simulink model "LKATestBenchExampleRL"  (R2020b)
settings: Solver=VariableStepAuto  StartTime=0.0  StopTime=simStopTime  RelTol=1e-3
PostLoadFcn:
  | helperLKASetUp
undefined symbols (not defined in the file): Curvature, CurvatureDerivative, DiscIntNeverNeededParam, driving, HeadingAngle, LateralOffset, Left, lr, m, PredictionHorizon, Right, Strength, Ts, v0_ego, yaw0_ego
libraries: simulink x4, drivingscenarioandsensors x2, mpcadaslib x1, rllib x1, autolibshared x1
CloseFcn:
  | helperLKACleanUp
settings Model: Creator=The MathWorks, Inc.  LastModifiedBy=adelicia
settings DataIOCC: ReturnWorkspaceOutputs=off
settings DebuggingCC: ParameterPrecisionLossMsg=none  ArithmeticOperatorsInVariantConditions=warning
settings HardwareCC: ProdLongLongMode=on
settings SFSimCC: SimUseLocalCustomCode=off
settings RTWCC: RTWUseLocalCustomCode=off

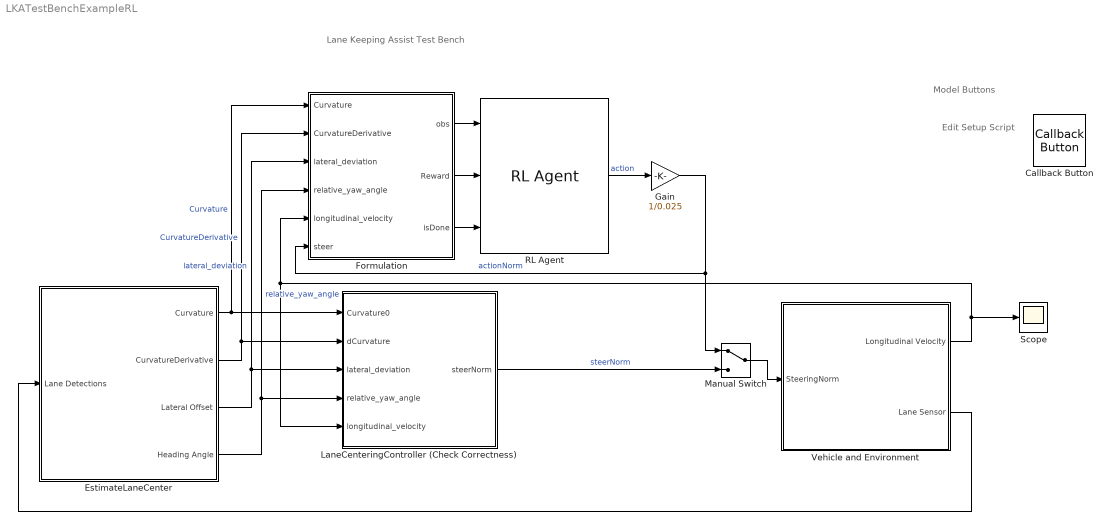
== system LKATestBenchExampleRL ==
  note: Edit Setup Script
  note: Lane Keeping Assist Test Bench
  note: Model Buttons
  Callback Button : CallbackButton  ButtonText=?
      settings: ClickFcn=|
      | exampleID = 'LaneKeepingAssistWithLaneDetectionExample';
      | exampleName = 'lane-keeping-assist-with-lane-detection.html';
      | if license('test','automated_driving_toolbox') && ~isempty(ver('driving'))
      |     helpview('driving',exampleID);
      | elseif license('test','MPC_Toolbox') && ~isempty(ver('mpc'))
      |     helpview('mpc',exampleID);
      | else
      |     web(fullfile('https://www.mathworks.com/help','driving','examples',exampleName));
      | end
      | clear exampleName exampleID;
  EstimateLaneCenter : Subsystem  VariantControl=v2
  Formulation : Subsystem
  Gain : Gain  Gain=1/0.025
  LaneCenteringController (Check Correctness) : Subsystem
  Manual Switch : ManualSwitch
  RL Agent : rllib/RL Agent  Agent=agent  ProvideReward=on  ProvideIsDone=on  ProvideCumRwd=off  TreatAsDirectFeedthrough=on  CollectLoggedSignals=on  CollectModelStates=on
  Scope : Scope
  Vehicle and Environment : Subsystem
  wires:
  Vehicle and Environment/2(Lane Sensor) -> EstimateLaneCenter/1(Lane Detections)
  EstimateLaneCenter/2(CurvatureDerivative) -> Formulation/2(CurvatureDerivative), LaneCenteringController (Check Correctness)/2(dCurvature)  "CurvatureDerivative"
  EstimateLaneCenter/3(Lateral Offset) -> Formulation/3(lateral_deviation), LaneCenteringController (Check Correctness)/3(lateral_deviation)  "lateral_deviation"
  EstimateLaneCenter/4(Heading Angle) -> Formulation/4(relative_yaw_angle), LaneCenteringController (Check Correctness)/4(relative_yaw_angle)  "relative_yaw_angle"
  Vehicle and Environment/1(Longitudinal Velocity) -> Scope/1, LaneCenteringController (Check Correctness)/5(longitudinal_velocity), Formulation/5(longitudinal_velocity)
  EstimateLaneCenter/1(Curvature) -> Formulation/1(Curvature), LaneCenteringController (Check Correctness)/1(Curvature0)  "Curvature"
  Formulation/1(obs) -> RL Agent/1
  Formulation/2(Reward) -> RL Agent/2
  Formulation/3(isDone) -> RL Agent/3
  LaneCenteringController (Check Correctness)/1(steerNorm) -> Manual Switch/2  "steerNorm"
  RL Agent/1 -> Gain/1  "action"
  Gain/1 -> Manual Switch/1, Formulation/6(steer)  "actionNorm"
  Manual Switch/1 -> Vehicle and Environment/1(SteeringNorm)

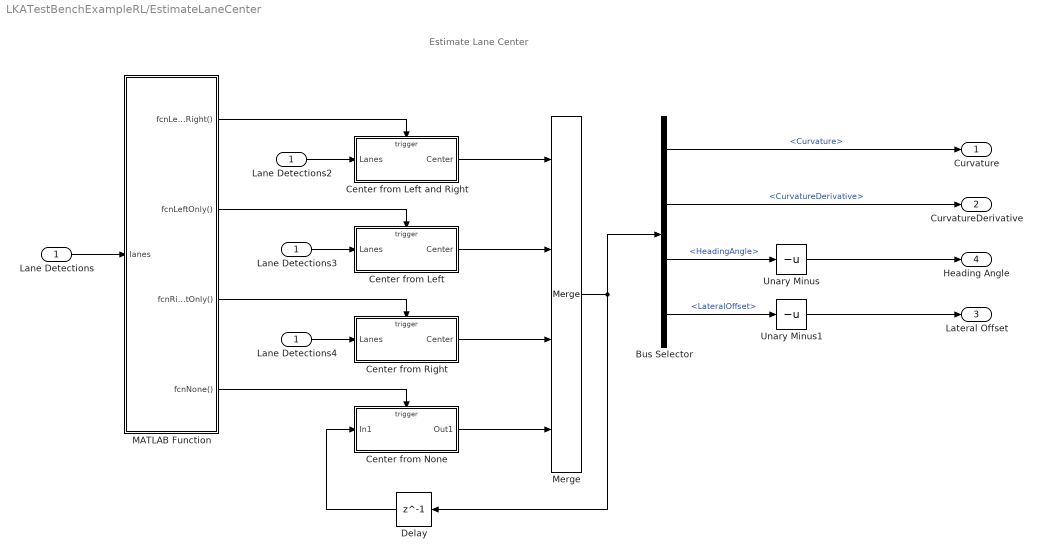
== system LKATestBenchExampleRL/EstimateLaneCenter ==
  note: Estimate Lane Center
  Lane Detections : Inport
  Bus Selector : BusSelector  OutputSignals=Curvature,CurvatureDerivative,HeadingAngle,LateralOffset
  Center from Left : Subsystem  TreatAsAtomicUnit=on
  Center from Left and Right : Subsystem  TreatAsAtomicUnit=on
  Center from None : Subsystem  TreatAsAtomicUnit=on
  Center from Right : Subsystem  TreatAsAtomicUnit=on
  Delay : Delay  DelayLength=1
  Lane Detections2 : InportShadow
  Lane Detections3 : InportShadow
  Lane Detections4 : InportShadow
  MATLAB Function : MATLAB Function  TreatAsAtomicUnit=on
  Merge : Merge  Inputs=4
  Unary Minus : UnaryMinus
  Unary Minus1 : UnaryMinus
  Curvature : Outport  VectorParamsAs1DForOutWhenUnconnected=off
  CurvatureDerivative : Outport  Port=2  VectorParamsAs1DForOutWhenUnconnected=off
  Lateral Offset : Outport  Port=3  VectorParamsAs1DForOutWhenUnconnected=off
  Heading Angle : Outport  Port=4  VectorParamsAs1DForOutWhenUnconnected=off
  wires:
  Bus Selector/3 -> Unary Minus/1  "<HeadingAngle>"
  Bus Selector/4 -> Unary Minus1/1  "<LateralOffset>"
  Bus Selector/1 -> Curvature/1  "<Curvature>"
  Bus Selector/2 -> CurvatureDerivative/1  "<CurvatureDerivative>"
  Unary Minus1/1 -> Lateral Offset/1
  Unary Minus/1 -> Heading Angle/1
  Merge/1 -> Delay/1, Bus Selector/1
  Center from Left/1(Center) -> Merge/2
  MATLAB Function/4(fcnNone()) -> Center from None/Trigger
  MATLAB Function/3(fcnRightOnly()) -> Center from Right/Trigger
  Lane Detections2/1 -> Center from Left and Right/1(Lanes)
  Lane Detections/1 -> MATLAB Function/1(lanes)
  Center from Left and Right/1(Center) -> Merge/1
  Delay/1 -> Center from None/1(In1)
  MATLAB Function/1(fcnLeftAndRight()) -> Center from Left and Right/Trigger
  Center from None/1(Out1) -> Merge/4
  MATLAB Function/2(fcnLeftOnly()) -> Center from Left/Trigger
  Lane Detections4/1 -> Center from Right/1(Lanes)
  Lane Detections3/1 -> Center from Left/1(Lanes)
  Center from Right/1(Center) -> Merge/3

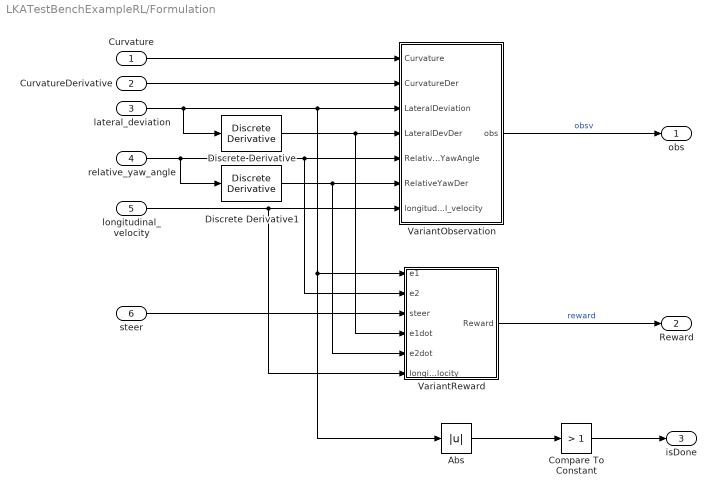
== system LKATestBenchExampleRL/Formulation ==
  Curvature : Inport
  CurvatureDerivative : Inport  Port=2
  lateral_deviation : Inport  Port=3
  relative_yaw_angle : Inport  Port=4
  longitudinal_velocity : Inport  Port=5
  steer : Inport  Port=6
  Abs : Abs
  Compare To Constant : simulink/Logic and Bit Operations/Compare To Constant  relop=>  const=1  OutDataTypeStr=boolean
  Discrete Derivative : simulink/Discrete/Discrete Derivative  gainval=1.0  ICPrevScaledInput=0.0  OutMin=[]  OutMax=[]  OutDataType=fixdt(1, 16)  OutScaling=2^-10  DoSatur=off
  Discrete Derivative1 : simulink/Discrete/Discrete Derivative  gainval=1.0  ICPrevScaledInput=0.0  OutMin=[]  OutMax=[]  OutDataType=fixdt(1, 16)  OutScaling=2^-10  DoSatur=off
  VariantObservation : Subsystem  Variant=on
  VariantReward : Subsystem  Variant=on
  obs : Outport
  Reward : Outport  Port=2  VectorParamsAs1DForOutWhenUnconnected=off
  isDone : Outport  Port=3  VectorParamsAs1DForOutWhenUnconnected=off
  wires:
  Curvature/1 -> VariantObservation/1(Curvature)
  CurvatureDerivative/1 -> VariantObservation/2(CurvatureDer)
  relative_yaw_angle/1 -> Discrete Derivative1/1, VariantReward/2(e2), VariantObservation/5(RelativeYawAngle)
  VariantObservation/1(obs) -> obs/1  "obsv"
  steer/1 -> VariantReward/3(steer)
  VariantReward/1(Reward) -> Reward/1  "reward"
  lateral_deviation/1 -> Discrete Derivative/1, Abs/1, VariantReward/1(e1), VariantObservation/3(LateralDeviation)
  Abs/1 -> Compare To Constant/1
  Compare To Constant/1 -> isDone/1
  Discrete Derivative/1 -> VariantReward/4(e1dot), VariantObservation/4(LateralDevDer)
  Discrete Derivative1/1 -> VariantReward/5(e2dot), VariantObservation/6(RelativeYawDer)
  longitudinal_velocity/1 -> VariantReward/6(longitudinal_velocity), VariantObservation/7(longitudinal_velocity)

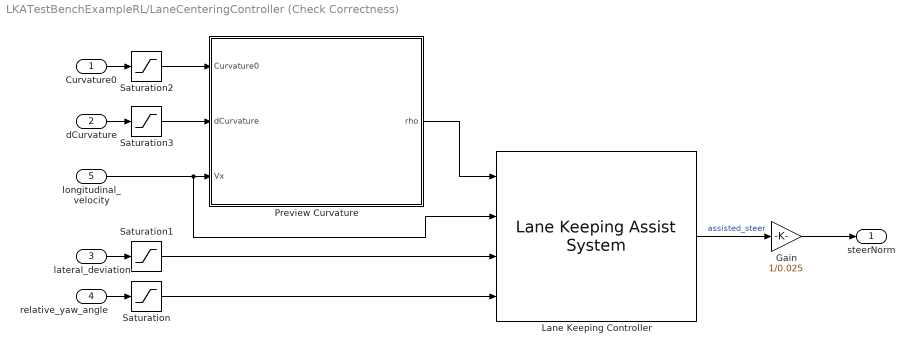
== system LKATestBenchExampleRL/LaneCenteringController (Check Correctness) ==
  Curvature0 : Inport
  dCurvature : Inport  Port=2
  lateral_deviation : Inport  Port=3
  relative_yaw_angle : Inport  Port=4
  longitudinal_velocity : Inport  Port=5
  Gain : Gain  Gain=1/0.025
  Lane Keeping Controller : mpcadaslib/Lane Keeping Assist System  ModelType=Use vehicle parameters  VehicleMass=m  VehicleYawInertia=Iz  LengthToFront=lf  LengthToRear=lr  FrontTireStiffness=Cf  RearTireStiffness=Cr  EgoModelMatrixA=[-4.4021 ,-12.4603;1.3913,-5.1868]  EgoModelMatrixB=[24.1270;15.8609]  EgoModelMatrixC=[1,0;0,1]  InitialLongVel=v0_ego  TransportLag=0  MinSteering=-0.5  umin_ext=off  MaxSteering=0.5  umax_ext=off  Ts=Ts  PredictionHorizon=PredictionHorizon  ControllerBehavior=0.200  suboptimal=off  maxiter=10  datatypeopt=single  optmode=off  trackmode=off
      settings: SourceProductBaseCode=MP
  Preview Curvature : MATLAB Function  TreatAsAtomicUnit=on  SystemSampleTime=Ts
  Saturation : Saturate
  Saturation1 : Saturate  UpperLimit=0.6  LowerLimit=-0.6
  Saturation2 : Saturate  UpperLimit=0.15  LowerLimit=-0.15
  Saturation3 : Saturate  UpperLimit=0.06  LowerLimit=-0.06
  steerNorm : Outport
  wires:
  relative_yaw_angle/1 -> Saturation/1
  dCurvature/1 -> Saturation3/1
  Preview Curvature/1(rho) -> Lane Keeping Controller/1
  longitudinal_velocity/1 -> Lane Keeping Controller/2, Preview Curvature/3(Vx)
  Curvature0/1 -> Saturation2/1
  lateral_deviation/1 -> Saturation1/1
  Saturation2/1 -> Preview Curvature/1(Curvature0)
  Saturation3/1 -> Preview Curvature/2(dCurvature)
  Saturation1/1 -> Lane Keeping Controller/3
  Saturation/1 -> Lane Keeping Controller/4
  Lane Keeping Controller/1 -> Gain/1  "assisted_steer"
  Gain/1 -> steerNorm/1

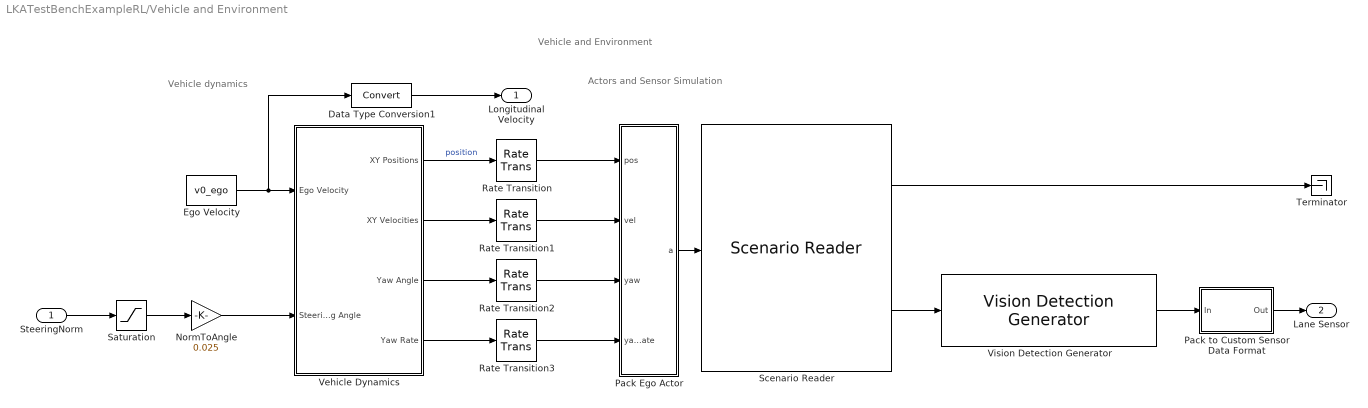
== system LKATestBenchExampleRL/Vehicle and Environment ==
  note: Vehicle dynamics
  note: Actors and Sensor Simulation
  note: Vehicle and Environment
  SteeringNorm : Inport  Unit=rad
  Data Type Conversion1 : DataTypeConversion
  Ego Velocity : Constant  Value=v0_ego  SampleTime=Ts
  NormToAngle : Gain  Gain=0.025
  Pack Ego Actor : MATLAB Function  TreatAsAtomicUnit=on
  Pack to Custom Sensor Data Format : Subsystem
  Rate Transition{,1..3} (4 alike) : RateTransition  OutPortSampleTime=Ts
  Saturation : Saturate  UpperLimit=1  LowerLimit=-1
  Scenario Reader : drivingscenarioandsensors/Scenario Reader  ScenarioSource=From workspace  ScenarioFileName=LKATestBenchScenario.mat  ScenarioVariableName=scenario  OutputCoordinateSystem=Vehicle coordinates  EgoVehicleSource=Input port  EgoVehicleActorID=1  OrientVehiclesOnRoad=off  OutputEgoVehiclePose=off  SampleTime=0.1  LaneBoundaryOutput=Ego vehicle lane boundaries  LaneBoundaryDistance=0:0.5:60  LaneBoundaryLocation=Inner edge of lane markings  BusNameSource=Auto  BusName=BusActors  BusName2Source=Auto  BusName2=BusLaneBoundaries  BusName3Source=Auto  BusName3=BusEgoActor  ShowCoordinateLabels=on  SimulateUsing=Interpreted execution
  Terminator : Terminator
  Vehicle Dynamics : Subsystem  VariantControl=VariantVDBS
  Vision Detection Generator : drivingscenarioandsensors/Vision Detection Generator  SensorIndex=1  DetectorOutput=Lanes only  UpdateInterval=0.1  LaneUpdateInterval=0.1  SensorLocation=[ 1.9, 0 ]  Height=1.1  Yaw=0  Pitch=1  Roll=0  BusNameSource=Auto  BusName=BusObjectDetections  BusName2Source=Property  BusName2=BusVision  MaxNumDetectionsSource=Property  MaxNumDetections=50  MaxNumLanesSource=Property  MaxNumLanes=2  DetectionCoordinates=Ego Cartesian  SimulateUsing=Interpreted execution  MaxRange=150  BoundingBoxAccuracy=5  ProcessNoiseIntensity=5  MaxSpeed=50  MaxAllowedOcclusion=0.5  MinObjectImageSize=[ 15, 15 ]  DetectionProbability=0.9  FalsePositivesPerImage=0.1  MinLaneImageSize=[ 20, 3 ]  LaneBoundaryAccuracy=3  HasNoise=on  InitialSeedSource=Repeatable  InitialSeed=0  UsedSeed=driving.internal.SimulinkUtilities.seedManager(gcb)  ActorProfilesSource=Parameters  ActorProfilesParameters=driving.internal.ActorProfilesParameters  ActorProfilesExpression=struct( 'ClassID', 0, 'Length', 4.7, 'Width', 1.8, 'Height', 1.4, 'OriginOffset', [ -1.35, 0, 0 ] )  Intrinsics=driving.internal.cameraIntrinsics
  Longitudinal Velocity : Outport  OutDataTypeStr=single  Unit=m/s  VectorParamsAs1DForOutWhenUnconnected=off
  Lane Sensor : Outport  Port=2  VectorParamsAs1DForOutWhenUnconnected=off
  wires:
  Ego Velocity/1 -> Data Type Conversion1/1, Vehicle Dynamics/1(Ego Velocity)
  Scenario Reader/1 -> Terminator/1
  Pack Ego Actor/1(a) -> Scenario Reader/1
  Vehicle Dynamics/2(XY Velocities) -> Rate Transition1/1
  Vehicle Dynamics/3(Yaw Angle) -> Rate Transition2/1
  Rate Transition/1 -> Pack Ego Actor/1(pos)
  Vehicle Dynamics/4(Yaw Rate) -> Rate Transition3/1
  Rate Transition2/1 -> Pack Ego Actor/3(yaw)
  Rate Transition1/1 -> Pack Ego Actor/2(vel)
  Rate Transition3/1 -> Pack Ego Actor/4(yawRate)
  Scenario Reader/2 -> Vision Detection Generator/1
  Vehicle Dynamics/1(XY Positions) -> Rate Transition/1  "position"
  Vision Detection Generator/1 -> Pack to Custom Sensor Data Format/1(In)
  Pack to Custom Sensor Data Format/1(Out) -> Lane Sensor/1
  Data Type Conversion1/1 -> Longitudinal Velocity/1
  SteeringNorm/1 -> Saturation/1
  NormToAngle/1 -> Vehicle Dynamics/2(Steering Angle)
  Saturation/1 -> NormToAngle/1

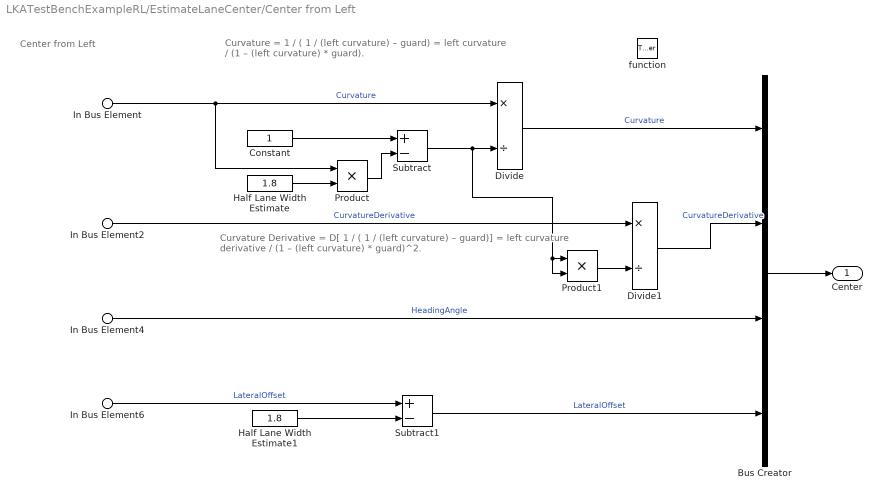
== system LKATestBenchExampleRL/EstimateLaneCenter/Center from Left ==
  note: Curvature
      | = 1 / ( 1 / (left curvature) – guard)
      | = left curvature / (1 – (left curvature) * guard).
  note: Center from Left
  note: Curvature Derivative
      | = D[ 1 / ( 1 / (left curvature) – guard)]
      | = left curvature derivative / (1 – (left curvature) * guard)^2.
  In Bus Element : Inport  PortName=Lanes  Element=Left.Curvature
  In Bus Element2 : Inport  PortName=Lanes  Element=Left.CurvatureDerivative
  In Bus Element4 : Inport  PortName=Lanes  Element=Left.HeadingAngle
  In Bus Element6 : Inport  PortName=Lanes  Element=Left.LateralOffset
  function : TriggerPort  TriggerType=function-call  VariantControl=Variant
  Bus Creator : BusCreator  Inputs=4
  Constant : Constant  OutDataTypeStr=Inherit: Inherit via back propagation
  Divide : Product  Inputs=*/
  Divide1 : Product  Inputs=*/
  Half Lane Width Estimate : Constant  Value=1.8  OutDataTypeStr=Inherit: Inherit via back propagation
  Half Lane Width Estimate1 : Constant  Value=1.8  OutDataTypeStr=Inherit: Inherit via back propagation
  Product : Product
  Product1 : Product
  Subtract : Sum  Inputs=+-
  Subtract1 : Sum  Inputs=+-
  Center : Outport  VectorParamsAs1DForOutWhenUnconnected=off
  wires:
  Bus Creator/1 -> Center/1
  Divide1/1 -> Bus Creator/2  "CurvatureDerivative"
  Divide/1 -> Bus Creator/1  "Curvature"
  In Bus Element4/1 -> Bus Creator/3  "HeadingAngle"
  Subtract1/1 -> Bus Creator/4  "LateralOffset"
  In Bus Element/1 -> Product/1, Divide/1  "Curvature"
  Subtract/1 -> Product1/2, Product1/1, Divide/2
  Half Lane Width Estimate/1 -> Product/2
  Constant/1 -> Subtract/1
  In Bus Element2/1 -> Divide1/1  "CurvatureDerivative"
  Product1/1 -> Divide1/2
  In Bus Element6/1 -> Subtract1/1  "LateralOffset"
  Half Lane Width Estimate1/1 -> Subtract1/2
  Product/1 -> Subtract/2

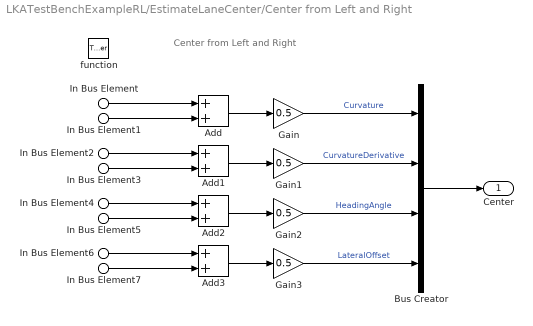
== system LKATestBenchExampleRL/EstimateLaneCenter/Center from Left and Right ==
  note: Center from Left and Right
  In Bus Element : Inport  PortName=Lanes  Element=Left.Curvature
  In Bus Element2 : Inport  PortName=Lanes  Element=Left.CurvatureDerivative
  In Bus Element4 : Inport  PortName=Lanes  Element=Left.HeadingAngle
  In Bus Element6 : Inport  PortName=Lanes  Element=Left.LateralOffset
  In Bus Element1 : Inport  PortName=Lanes  Element=Right.Curvature
  In Bus Element3 : Inport  PortName=Lanes  Element=Right.CurvatureDerivative
  In Bus Element5 : Inport  PortName=Lanes  Element=Right.HeadingAngle
  In Bus Element7 : Inport  PortName=Lanes  Element=Right.LateralOffset
  function : TriggerPort  TriggerType=function-call  VariantControl=Variant
  Add{,1..3} (4 alike) : Sum
  Bus Creator : BusCreator  Inputs=4
  Gain{,1..3} (4 alike) : Gain  Gain=0.5
  Center : Outport  VectorParamsAs1DForOutWhenUnconnected=off
  wires:
  Add/1 -> Gain/1
  Gain/1 -> Bus Creator/1  "Curvature"
  Add1/1 -> Gain1/1
  Gain1/1 -> Bus Creator/2  "CurvatureDerivative"
  Add2/1 -> Gain2/1
  Gain2/1 -> Bus Creator/3  "HeadingAngle"
  Add3/1 -> Gain3/1
  Gain3/1 -> Bus Creator/4  "LateralOffset"
  Bus Creator/1 -> Center/1
  In Bus Element/1 -> Add/1
  In Bus Element1/1 -> Add/2
  In Bus Element2/1 -> Add1/1
  In Bus Element3/1 -> Add1/2
  In Bus Element4/1 -> Add2/1
  In Bus Element5/1 -> Add2/2
  In Bus Element7/1 -> Add3/2
  In Bus Element6/1 -> Add3/1

== system LKATestBenchExampleRL/EstimateLaneCenter/Center from None ==
  In1 : Inport
  function : TriggerPort  TriggerType=function-call  VariantControl=Variant
  Out1 : Outport  VectorParamsAs1DForOutWhenUnconnected=off
  wires:
  In1/1 -> Out1/1

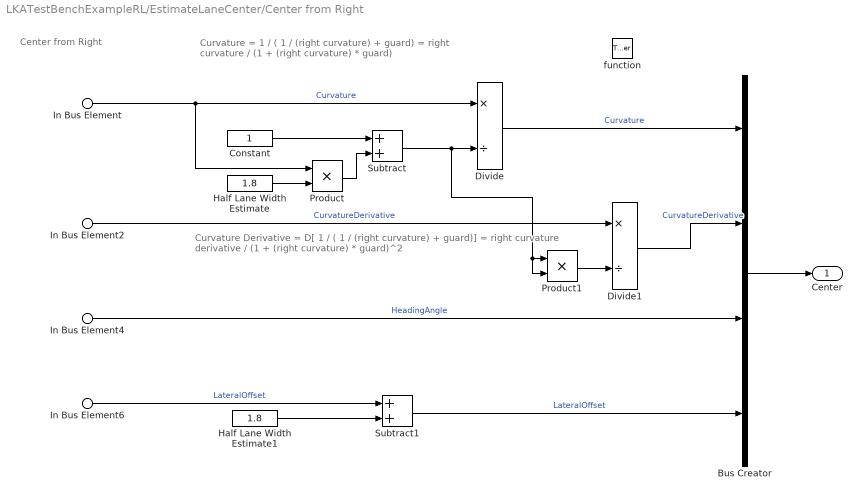
== system LKATestBenchExampleRL/EstimateLaneCenter/Center from Right ==
  note: Center from Right
  note: Curvature
      | = 1 / ( 1 / (right curvature) + guard)
      | = right curvature / (1 + (right curvature) * guard)
  note: Curvature Derivative
      | = D[ 1 / ( 1 / (right curvature) + guard)]
      | = right curvature derivative / (1 + (right curvature) * guard)^2
  In Bus Element : Inport  PortName=Lanes  Element=Right.Curvature
  In Bus Element2 : Inport  PortName=Lanes  Element=Right.CurvatureDerivative
  In Bus Element4 : Inport  PortName=Lanes  Element=Right.HeadingAngle
  In Bus Element6 : Inport  PortName=Lanes  Element=Right.LateralOffset
  function : TriggerPort  TriggerType=function-call  VariantControl=Variant
  Bus Creator : BusCreator  Inputs=4
  Constant : Constant  OutDataTypeStr=Inherit: Inherit via back propagation
  Divide : Product  Inputs=*/
  Divide1 : Product  Inputs=*/
  Half Lane Width Estimate : Constant  Value=1.8  OutDataTypeStr=Inherit: Inherit via back propagation
  Half Lane Width Estimate1 : Constant  Value=1.8  OutDataTypeStr=Inherit: Inherit via back propagation
  Product : Product
  Product1 : Product
  Subtract : Sum
  Subtract1 : Sum
  Center : Outport  VectorParamsAs1DForOutWhenUnconnected=off
  wires:
  In Bus Element2/1 -> Divide1/1  "CurvatureDerivative"
  Divide1/1 -> Bus Creator/2  "CurvatureDerivative"
  Product1/1 -> Divide1/2
  In Bus Element4/1 -> Bus Creator/3  "HeadingAngle"
  Half Lane Width Estimate1/1 -> Subtract1/2
  In Bus Element6/1 -> Subtract1/1  "LateralOffset"
  Divide/1 -> Bus Creator/1  "Curvature"
  Subtract1/1 -> Bus Creator/4  "LateralOffset"
  Bus Creator/1 -> Center/1
  In Bus Element/1 -> Product/1, Divide/1  "Curvature"
  Subtract/1 -> Product1/2, Product1/1, Divide/2
  Constant/1 -> Subtract/1
  Product/1 -> Subtract/2
  Half Lane Width Estimate/1 -> Product/2

== system LKATestBenchExampleRL/Formulation/VariantObservation ==
  note: 1) Add Subsystem or Model blocks as valid variant choices.
      | 2) You cannot connect blocks at this level. At simulation, connectivity is automatically
      | determined, based on the active variant and port name matching.
  Curvature : Inport
  CurvatureDer : Inport  Port=2
  LateralDeviation : Inport  Port=3
  LateralDevDer : Inport  Port=4
  RelativeYawAngle : Inport  Port=5
  RelativeYawDer : Inport  Port=6
  longitudinal_velocity : Inport  Port=7
  EightStates : Subsystem  VariantControl=OBSV_MODE_EIGHT
  FourStates : Subsystem  VariantControl=OBSV_MODE_FOUR
  TwoStates : Subsystem  VariantControl=OBSV_MODE_TWO
  obs : Outport

== system LKATestBenchExampleRL/Formulation/VariantReward ==
  note: 1) Add Subsystem or Model blocks as valid variant choices.
      | 2) You cannot connect blocks at this level. At simulation, connectivity is automatically
      | determined, based on the active variant and port name matching.
  e1 : Inport
  e2 : Inport  Port=2
  steer : Inport  Port=3
  e1dot : Inport  Port=4
  e2dot : Inport  Port=5
  longitudinal_velocity : Inport  Port=6
  QuardraticReward : Subsystem  VariantControl=REWARD_MODE_QUADRATIC
  TrgonometryReward : Subsystem  VariantControl=REWARD_MODE_TRIGONOMETRY
  Reward : Outport

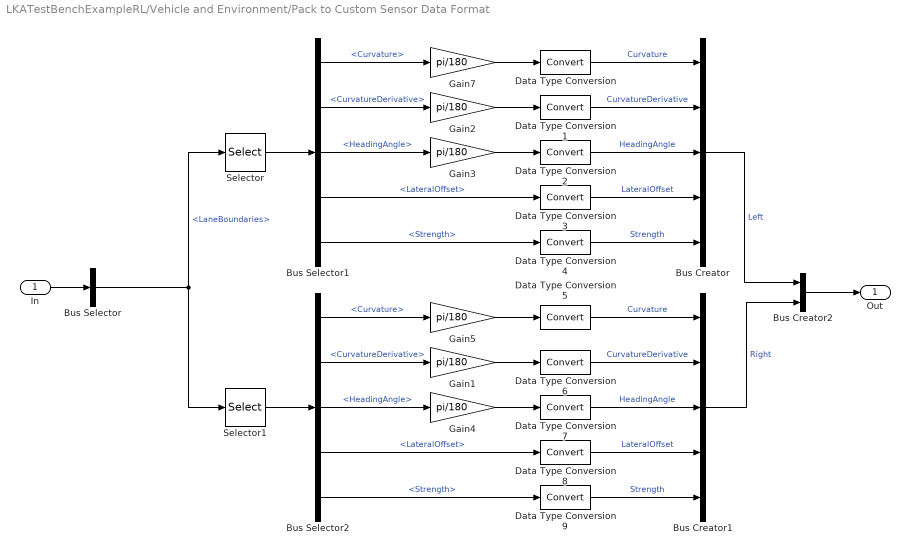
== system LKATestBenchExampleRL/Vehicle and Environment/Pack to Custom Sensor Data Format ==
  In : Inport
  Bus Creator : BusCreator  Inputs=Curvature,CurvatureDerivative,HeadingAngle,LateralOffset,Strength  OutDataTypeStr=Bus: LaneSensorBoundaries
  Bus Creator1 : BusCreator  Inputs=Curvature,CurvatureDerivative,HeadingAngle,LateralOffset,Strength  OutDataTypeStr=Bus: LaneSensorBoundaries
  Bus Creator2 : BusCreator  Inputs=Left,Right  OutDataTypeStr=Bus: LaneSensor
  Bus Selector : BusSelector  OutputSignals=LaneBoundaries
  Bus Selector1 : BusSelector  OutputSignals=Curvature,CurvatureDerivative,HeadingAngle,LateralOffset,Strength
  Bus Selector2 : BusSelector  OutputSignals=Curvature,CurvatureDerivative,HeadingAngle,LateralOffset,Strength
  Data Type Conversion{,1..9} (10 alike) : DataTypeConversion
  Gain{1..5,7} (6 alike) : Gain  Gain=pi/180
  Selector : Selector  InputPortWidth=2  IndexOptions=Index vector (dialog)  Indices=1  OutputSizes=1
  Selector1 : Selector  InputPortWidth=2  IndexOptions=Index vector (dialog)  Indices=2  OutputSizes=1
  Out : Outport  VectorParamsAs1DForOutWhenUnconnected=off
  wires:
  In/1 -> Bus Selector/1
  Bus Selector/1 -> Selector/1, Selector1/1  "<LaneBoundaries>"
  Selector/1 -> Bus Selector1/1
  Bus Selector1/2 -> Gain2/1  "<CurvatureDerivative>"
  Bus Selector1/1 -> Gain7/1  "<Curvature>"
  Bus Selector1/3 -> Gain3/1  "<HeadingAngle>"
  Gain7/1 -> Data Type Conversion/1
  Gain2/1 -> Data Type Conversion1/1
  Gain3/1 -> Data Type Conversion2/1
  Bus Selector1/4 -> Data Type Conversion3/1  "<LateralOffset>"
  Bus Selector1/5 -> Data Type Conversion4/1  "<Strength>"
  Data Type Conversion/1 -> Bus Creator/1  "Curvature"
  Data Type Conversion1/1 -> Bus Creator/2  "CurvatureDerivative"
  Data Type Conversion2/1 -> Bus Creator/3  "HeadingAngle"
  Data Type Conversion3/1 -> Bus Creator/4  "LateralOffset"
  Data Type Conversion4/1 -> Bus Creator/5  "Strength"
  Data Type Conversion9/1 -> Bus Creator1/5  "Strength"
  Data Type Conversion6/1 -> Bus Creator1/2  "CurvatureDerivative"
  Data Type Conversion7/1 -> Bus Creator1/3  "HeadingAngle"
  Data Type Conversion8/1 -> Bus Creator1/4  "LateralOffset"
  Data Type Conversion5/1 -> Bus Creator1/1  "Curvature"
  Bus Selector2/1 -> Gain5/1  "<Curvature>"
  Selector1/1 -> Bus Selector2/1
  Bus Selector2/4 -> Data Type Conversion8/1  "<LateralOffset>"
  Bus Selector2/5 -> Data Type Conversion9/1  "<Strength>"
  Bus Selector2/2 -> Gain1/1  "<CurvatureDerivative>"
  Gain4/1 -> Data Type Conversion7/1
  Gain5/1 -> Data Type Conversion5/1
  Gain1/1 -> Data Type Conversion6/1
  Bus Selector2/3 -> Gain4/1  "<HeadingAngle>"
  Bus Creator2/1 -> Out/1
  Bus Creator/1 -> Bus Creator2/1  "Left"
  Bus Creator1/1 -> Bus Creator2/2  "Right"

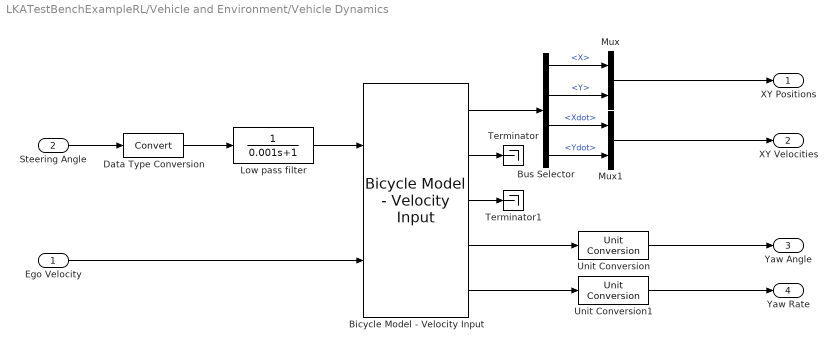
== system LKATestBenchExampleRL/Vehicle and Environment/Vehicle Dynamics ==
  Ego Velocity : Inport
  Steering Angle : Inport  Port=2
  Bicycle Model - Velocity Input : autolibshared/Bicycle Model - Velocity Input  trackMode=Single (bicycle)  inputMode=External longitudinal forces  frontSteerMode=on  rearSteerMode=off  windMode=off  muMode=off  extFMode=off  extMMode=off  aMode=3  NF=2  NR=2  m=m  a=lf  b=lr  h=0.35  X_o=x0_ego  xdot_o=0  CalphaMode=off  sigmaMode=on  w=[1.4,1.4]  Cy_f=Cf  Cy_r=Cr  sigma_f=.1  sigma_r=.1  alpha_f_brk=[-.1 .1]  Cy_f_data=[-9e3 9e3]  alpha_r_brk=[-.1 .1]  Cy_r_data=[-9e3 9e3]  Y_o=y0_ego  ydot_o=0  Izz=Iz  psi_o=yaw0_ego*pi/180  r_o=0  Af=2  Cd=.3  Cl=.1  Cpm=.1  beta_w=[0:0.01:0.3]  Cs=[0:0.03:0.9]  Cym=[0:0.01:0.3]  Pabs=101325  Tair=273  g=9.81  mu=1  xdot_tol=.01  Fznom=5000  Fxtire_sat=1e6  Fytire_sat=1e6  longOff=0  latOff=0  vertOff=0
      settings: SourceProductBaseCode=PW,MT,UV,VE,VP
  Bus Selector : BusSelector  OutputSignals=InertFrm.FrntAxl.Disp.X,InertFrm.FrntAxl.Disp.Y,InertFrm.FrntAxl.Vel.Xdot,InertFrm.FrntAxl.Vel.Ydot
  Data Type Conversion : DataTypeConversion
  Low pass filter : TransferFcn  Denominator=[0.001 1]
  Mux : Mux  Inputs=2
  Mux1 : Mux  Inputs=2
  Terminator : Terminator
  Terminator1 : Terminator
  Unit Conversion : UnitConversion  OutputType=Inherit: Inherit via back propagation
  Unit Conversion1 : UnitConversion  OutputType=Inherit: Inherit via back propagation
  XY Positions : Outport  Unit=m  VectorParamsAs1DForOutWhenUnconnected=off
  XY Velocities : Outport  Port=2  Unit=m/s  VectorParamsAs1DForOutWhenUnconnected=off
  Yaw Angle : Outport  Port=3  Unit=deg  VectorParamsAs1DForOutWhenUnconnected=off
  Yaw Rate : Outport  Port=4  Unit=degree/s  VectorParamsAs1DForOutWhenUnconnected=off
  wires:
  Mux/1 -> XY Positions/1
  Mux1/1 -> XY Velocities/1
  Unit Conversion1/1 -> Yaw Rate/1
  Unit Conversion/1 -> Yaw Angle/1
  Ego Velocity/1 -> Bicycle Model - Velocity Input/2
  Bicycle Model - Velocity Input/1 -> Bus Selector/1
  Bicycle Model - Velocity Input/2 -> Terminator/1
  Bicycle Model - Velocity Input/3 -> Terminator1/1
  Bicycle Model - Velocity Input/4 -> Unit Conversion/1
  Bicycle Model - Velocity Input/5 -> Unit Conversion1/1
  Bus Selector/1 -> Mux/1  "<X>"
  Bus Selector/2 -> Mux/2  "<Y>"
  Bus Selector/3 -> Mux1/1  "<Xdot>"
  Bus Selector/4 -> Mux1/2  "<Ydot>"
  Data Type Conversion/1 -> Low pass filter/1
  Steering Angle/1 -> Data Type Conversion/1
  Low pass filter/1 -> Bicycle Model - Velocity Input/1

== system LKATestBenchExampleRL/Formulation/VariantObservation/EightStates ==
  Curvature : Inport
  CurvatureDer : Inport  Port=2
  LateralDeviation : Inport  Port=3
  LateralDevDer : Inport  Port=4
  RelativeYawAngle : Inport  Port=5
  RelativeYawDer : Inport  Port=6
  longitudinal_velocity : Inport  Port=7
  Discrete-Time Integrator : DiscreteIntegrator  SampleTime=-1  ICPrevOutput=DiscIntNeverNeededParam  ICPrevScaledInput=DiscIntNeverNeededParam
  Discrete-Time Integrator1 : DiscreteIntegrator  SampleTime=-1  ICPrevOutput=DiscIntNeverNeededParam  ICPrevScaledInput=DiscIntNeverNeededParam
  Mux : Mux  Inputs=8
  Terminator : Terminator
  obs : Outport  VectorParamsAs1DForOutWhenUnconnected=off
  wires:
  Mux/1 -> obs/1
  CurvatureDer/1 -> Mux/2
  Curvature/1 -> Mux/1
  LateralDeviation/1 -> Discrete-Time Integrator1/1, Mux/3
  Discrete-Time Integrator1/1 -> Mux/4  "integral_error"
  RelativeYawAngle/1 -> Discrete-Time Integrator/1, Mux/6
  Discrete-Time Integrator/1 -> Mux/7  "integral_error"
  LateralDevDer/1 -> Mux/5
  RelativeYawDer/1 -> Mux/8
  longitudinal_velocity/1 -> Terminator/1

== system LKATestBenchExampleRL/Formulation/VariantObservation/FourStates ==
  Curvature : Inport
  CurvatureDer : Inport  Port=2
  LateralDeviation : Inport  Port=3
  LateralDevDer : Inport  Port=4
  RelativeYawAngle : Inport  Port=5
  RelativeYawDer : Inport  Port=6
  longitudinal_velocity : Inport  Port=7
  Mux : Mux
  Terminator1 : Terminator
  Terminator2 : Terminator
  Terminator3 : Terminator
  obs : Outport  VectorParamsAs1DForOutWhenUnconnected=off
  wires:
  Mux/1 -> obs/1
  Curvature/1 -> Mux/1
  CurvatureDer/1 -> Mux/2
  LateralDevDer/1 -> Terminator1/1
  RelativeYawDer/1 -> Terminator2/1
  RelativeYawAngle/1 -> Mux/4
  LateralDeviation/1 -> Mux/3
  longitudinal_velocity/1 -> Terminator3/1

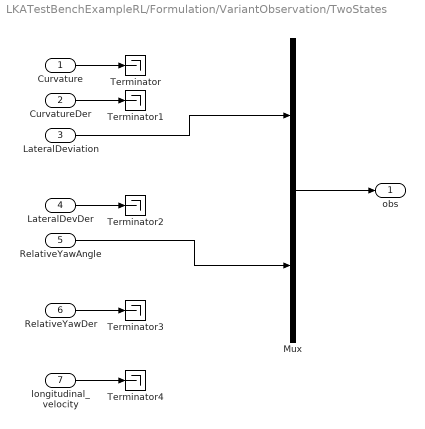
== system LKATestBenchExampleRL/Formulation/VariantObservation/TwoStates ==
  Curvature : Inport
  CurvatureDer : Inport  Port=2
  LateralDeviation : Inport  Port=3
  LateralDevDer : Inport  Port=4
  RelativeYawAngle : Inport  Port=5
  RelativeYawDer : Inport  Port=6
  longitudinal_velocity : Inport  Port=7
  Mux : Mux  Inputs=2
  Terminator{,1..4} (5 alike) : Terminator
  obs : Outport  VectorParamsAs1DForOutWhenUnconnected=off
  wires:
  Mux/1 -> obs/1
  Curvature/1 -> Terminator/1
  CurvatureDer/1 -> Terminator1/1
  LateralDeviation/1 -> Mux/1
  RelativeYawAngle/1 -> Mux/2
  LateralDevDer/1 -> Terminator2/1
  RelativeYawDer/1 -> Terminator3/1
  longitudinal_velocity/1 -> Terminator4/1

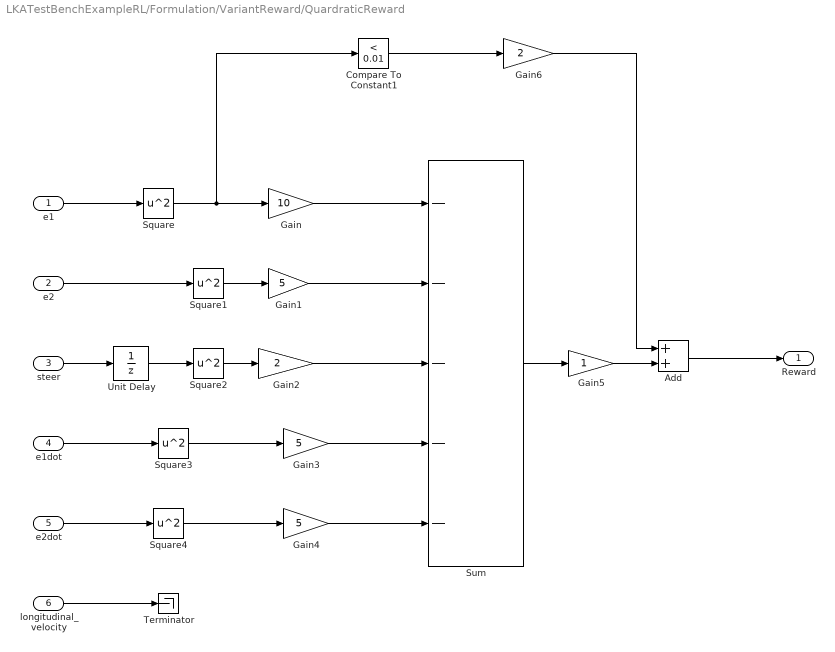
== system LKATestBenchExampleRL/Formulation/VariantReward/QuardraticReward ==
  e1 : Inport
  e2 : Inport  Port=2
  steer : Inport  Port=3
  e1dot : Inport  Port=4
  e2dot : Inport  Port=5
  longitudinal_velocity : Inport  Port=6
  Add : Sum
  Compare To Constant1 : simulink/Logic and Bit Operations/Compare To Constant  relop=<  const=0.01  OutDataTypeStr=boolean
  Gain : Gain  Gain=10
  Gain1 : Gain  Gain=5
  Gain2 : Gain  Gain=2
  Gain3 : Gain  Gain=5
  Gain4 : Gain  Gain=5
  Gain5 : Gain
  Gain6 : Gain  Gain=2
  Square{,1..4} (5 alike) : Math  Operator=square  SignedPower=on  SaturateOnIntegerOverflow=on
  Sum : Sum  Inputs=-----
  Terminator : Terminator
  Unit Delay : UnitDelay  SampleTime=-1  HasFrameUpgradeWarning=on
  Reward : Outport  VectorParamsAs1DForOutWhenUnconnected=off
  wires:
  Gain1/1 -> Sum/2
  e1/1 -> Square/1
  e2/1 -> Square1/1
  Sum/1 -> Gain5/1
  Gain/1 -> Sum/1
  Square1/1 -> Gain1/1
  steer/1 -> Unit Delay/1
  Square2/1 -> Gain2/1
  Gain2/1 -> Sum/3
  Unit Delay/1 -> Square2/1
  e2dot/1 -> Square4/1
  Square3/1 -> Gain3/1
  e1dot/1 -> Square3/1
  Square4/1 -> Gain4/1
  Gain3/1 -> Sum/4
  Gain4/1 -> Sum/5
  Gain5/1 -> Add/2
  Square/1 -> Compare To Constant1/1, Gain/1
  Compare To Constant1/1 -> Gain6/1
  Gain6/1 -> Add/1
  Add/1 -> Reward/1
  longitudinal_velocity/1 -> Terminator/1

== system LKATestBenchExampleRL/Formulation/VariantReward/TrgonometryReward ==
  note: annotation
  e1 : Inport
  e2 : Inport  Port=2
  steer : Inport  Port=3
  e1dot : Inport  Port=4
  e2dot : Inport  Port=5
  longitudinal_velocity : Inport  Port=6
  MATLAB Function : MATLAB Function  TreatAsAtomicUnit=on
  Terminator{,1..3} (4 alike) : Terminator
  Reward : Outport  VectorParamsAs1DForOutWhenUnconnected=off
  wires:
  e2dot/1 -> Terminator2/1
  e1dot/1 -> Terminator1/1
  MATLAB Function/1(r) -> Reward/1
  steer/1 -> Terminator/1
  e2/1 -> MATLAB Function/2(theta)
  e1/1 -> MATLAB Function/1(d)
  longitudinal_velocity/1 -> Terminator3/1

== matlab function LKATestBenchExampleRL/Formulation/VariantReward/TrgonometryReward/MATLAB Function ==
  data: d input; r output; theta input
function r = fcn(d, theta)
w = 1.8; % half width
if abs(theta) < pi/3 && abs(d) <w/2
    r = single(cos(theta)-0.5*sin(abs(theta))-d/w);
else
    r = single(-2);
end

end

== matlab function LKATestBenchExampleRL/Vehicle and Environment/Pack Ego Actor ==
  data: pos input; a output Bus: BusActors1Actors size=1; vel input; yaw input; yawRate input
function a = packEgo(pos,vel,yaw,yawRate)
% Pack ego information into a single ego actor bus
%
% Imoprtant note:
% Output is a bus of type BusActorsActors. This is the same bus used by the
% Scenario Reader to output an individual actor. If you change the
% output bus name of Scenario Reader change the output bus name here
% as well by clicking on 'Edit Data' in the menu above.

a = struct(...
    'ActorID',1,...
    'Position', [pos(1) pos(2) 0], ...
    'Velocity', [vel(1) vel(2) 0], ...
    'Roll', 0, ...
    'Pitch', 0, ...
    'Yaw', yaw, ...
    'AngularVelocity', [0 0 yawRate]);

== matlab function LKATestBenchExampleRL/EstimateLaneCenter/MATLAB Function ==
  data: lanes input
  events: fcnLeftAndRight output FUNCTION_CALL_EVENT; fcnLeftOnly output FUNCTION_CALL_EVENT; fcnRightOnly output FUNCTION_CALL_EVENT; fcnNone output FUNCTION_CALL_EVENT
function fcn(lanes)

leftStrength  = lanes.Left.Strength;
rightStrength = lanes.Right.Strength;

if (leftStrength > 0) && (rightStrength > 0)
   fcnLeftAndRight();
   
elseif leftStrength > 0
    fcnLeftOnly();
    
elseif rightStrength > 0
    fcnRightOnly();
    
else
    fcnNone();
end

== matlab function LKATestBenchExampleRL/LaneCenteringController (Check Correctness)/Preview Curvature ==
  data: rho output; Curvature0 input; dCurvature input; Vx input; Ts parameter; PredictionHorizon parameter
function rho = predictCurvature(Curvature0,dCurvature,Vx, Ts, PredictionHorizon)
% Curvature0 = initial curvature per unit length                  [1/m]
% dCurvature = (constant) derivative of curvature per unit length [1/m^2]
% CurvatureLength = length for which the clothoid model is valid [m]
% Vx = speed of vehicle

% We want to export a set of curvatures at a uniform sample time ahead.
% t is this vector which goes up to 1 second in the future or having
% enough time to reach the known length in curvature (whichever is smaller)

% To enable truncation by curvelength, mark output "rho" as varsize
%t = 0:Ts:min(1,CurvatureLength/Vx);

t = zeros(PredictionHorizon+1,1);
for i=1:numel(t)
    t(i) = (i-1).*Ts;
end

% We compute the curvature vector rho(t) using the specified clothoid model
rho = Curvature0 + dCurvature*Vx*t;
